simulink model "modelo_equivalente_mecanico"  (R2023b)
settings: Solver=VariableStepAuto  StartTime=0.0  StopTime=10.0  RelTol=1e-3
PreLoadFcn:
  | Jcm=0.0208;
values from neighbouring files (symbols this model uses):
  b_eq = b_m + b_l/(r^2)    (= 2.19444444444e-05)    [polos_y_ceros.m]    (also in var1.m)
  J_eq = J_m + J_l/(r^2)    (= 1.97847222222e-05)    [polos_y_ceros.m]    (also in var1.m = 4.58263888889e-05)
  L_d = 6.6 * 10^(-3)    (= 0.0066)    [polos_y_ceros.m]    (also in var1.m)
  L_q = 5.8 * 10^(-3)    (= 0.0058)    [polos_y_ceros.m]    (also in var1.m)
  lambda_m = 0.016    [polos_y_ceros.m]    (also in var1.m)
  P_p = 3    [polos_y_ceros.m]    (also in var1.m)
  r = 120/1    (= 120)    [polos_y_ceros.m]    (also in var1.m)
undefined symbols (not defined in the file or in its folder): bl
settings Model: Creator=tomas  LastModifiedBy=tomas

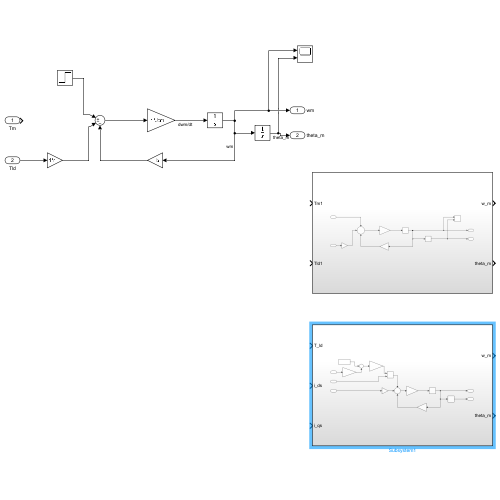
[thumbnail: Simulink's stored preview of the top-level diagram]
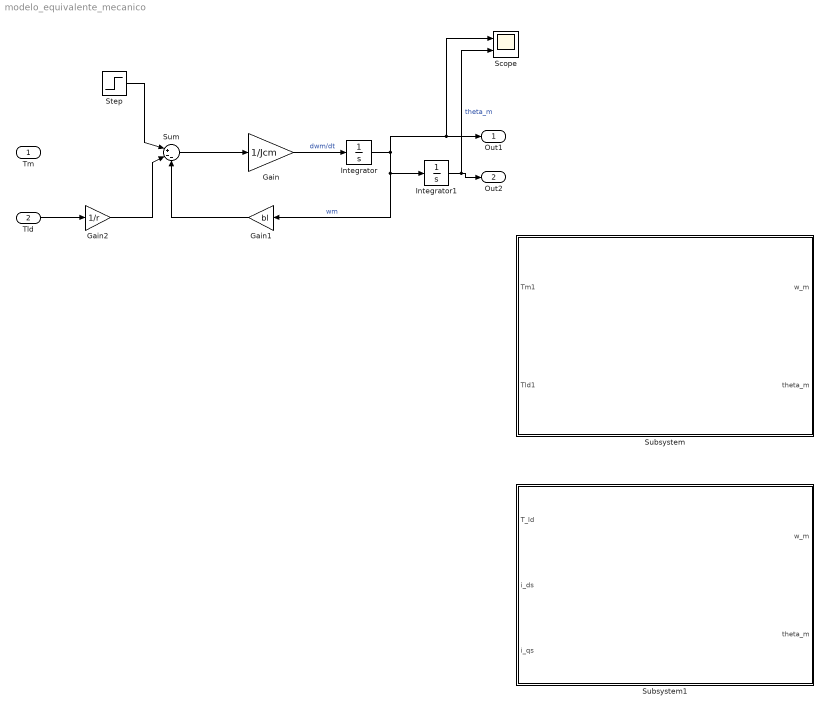
== system modelo_equivalente_mecanico ==
  Tm : Inport
  Tld : Inport  Port=2
  Gain : Gain  Gain=1/Jcm
  Gain1 : Gain  Gain=bl
  Gain2 : Gain  Gain=1/r
  Integrator : Integrator
  Integrator1 : Integrator
  Scope : Scope  NumInputPorts=2
  Step : Step  SampleTime=0
  Subsystem : Subsystem
  Subsystem1 : Subsystem
  Sum : Sum  Inputs=|+--
  Out1 : Outport  SignalName=wm
  Out2 : Outport  Port=2  SignalName=theta_m
  wires:
  Sum/1 -> Gain/1
  Gain/1 -> Integrator/1  "dwm/dt"
  Integrator/1 -> Integrator1/1, Gain1/1, Scope/1, Out1/1  "wm"
  Gain1/1 -> Sum/3
  Integrator1/1 -> Scope/2, Out2/1  "theta_m"
  Tld/1 -> Gain2/1
  Gain2/1 -> Sum/2
  Step/1 -> Sum/1

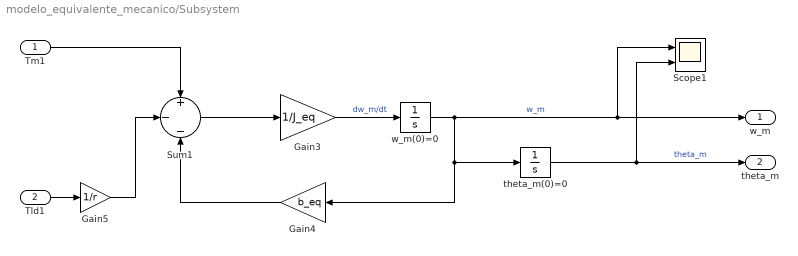
== system modelo_equivalente_mecanico/Subsystem ==
  Tm1 : Inport
  Tld1 : Inport  Port=2
  Gain3 : Gain  Gain=1/J_eq
  Gain4 : Gain  Gain=b_eq
  Gain5 : Gain  Gain=1/r
  Scope1 : Scope  NumInputPorts=2
  Sum1 : Sum  Inputs=+|-|-
  theta_m(0)=0 : Integrator
  w_m(0)=0 : Integrator
  w_m : Outport
  theta_m : Outport  Port=2
  wires:
  Tm1/1 -> Sum1/1
  Gain4/1 -> Sum1/3
  w_m(0)=0/1 -> theta_m(0)=0/1, Gain4/1, Scope1/1, w_m/1  "w_m"
  Sum1/1 -> Gain3/1
  Gain3/1 -> w_m(0)=0/1  "dw_m/dt"
  Tld1/1 -> Gain5/1
  theta_m(0)=0/1 -> Scope1/2, theta_m/1  "theta_m"
  Gain5/1 -> Sum1/2

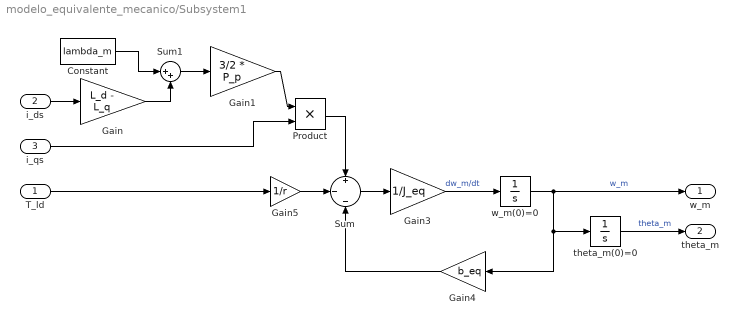
== system modelo_equivalente_mecanico/Subsystem1 ==
  T_ld : Inport
  i_ds : Inport  Port=2
  i_qs : Inport  Port=3
  Constant : Constant  Value=lambda_m
  Gain : Gain  Gain=L_d - L_q
  Gain1 : Gain  Gain=3/2 * P_p
  Gain3 : Gain  Gain=1/J_eq
  Gain4 : Gain  Gain=b_eq
  Gain5 : Gain  Gain=1/r
  Product : Product
  Sum : Sum  Inputs=+|-|-
  Sum1 : Sum  Inputs=|++
  theta_m(0)=0 : Integrator
  w_m(0)=0 : Integrator
  w_m : Outport
  theta_m : Outport  Port=2
  wires:
  w_m(0)=0/1 -> w_m/1, theta_m(0)=0/1, Gain4/1  "w_m"
  Sum/1 -> Gain3/1
  Gain3/1 -> w_m(0)=0/1  "dw_m/dt"
  T_ld/1 -> Gain5/1
  theta_m(0)=0/1 -> theta_m/1  "theta_m"
  i_ds/1 -> Gain/1
  Constant/1 -> Sum1/1
  Gain/1 -> Sum1/2
  Sum1/1 -> Gain1/1
  Gain1/1 -> Product/1
  i_qs/1 -> Product/2
  Product/1 -> Sum/1
  Gain4/1 -> Sum/3
  Gain5/1 -> Sum/2
